simulink model "ToySystem"  (R2019b)
settings: Solver=VariableStepAuto  StartTime=0.0  StopTime=10.0  RelTol=1e-3
undefined symbols (not defined in the file or in its folder): b1, b2, Cp_wall, D, dH, dH1, dH2, f, f1, f2, Fluid, Fluid1, Fluid2, H, HTC, HTC1, HTC2, HTC_method, HTC_method1, HTC_method2, KL, KL1, KL2, L, L1, L2, M_wall, Nu_lam1, Nu_lam2, P_init, PAF, Pamb, Pass1, Pass2, rev_comms_sink, Tw_init, v, W1, W2
libraries: DAEMOT_Lib x21
(part 1 of 2)
settings Model: Creator=aksland2  LastModifiedBy=aksland2

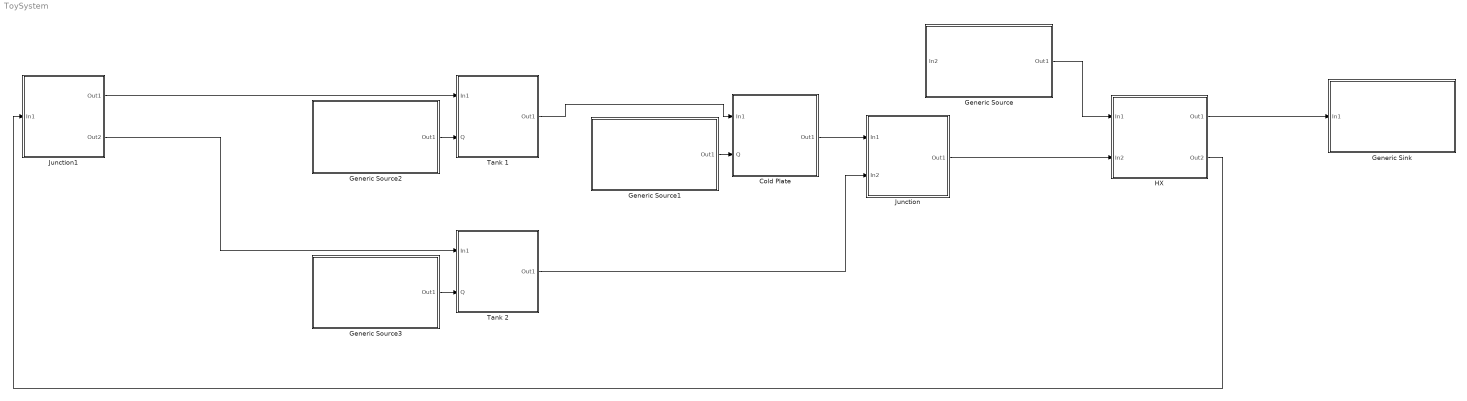
== system ToySystem ==
  Cold Plate : Subsystem  AncestorBlock=DAEMOT_Lib/Thermal/Cold_Plate  mask(Cold Plate){fluid=PG50, P_init=113, T_init=20, cp_f=4000}
      mask prompts: fluid "Fluid Type"; P_init "Initial Outlet Pressure [kPa]"; T_init "Initial Outlet Temperature [°C]"; cp_f "Specific Head"
      mask help: Tracks the time rate of change of the pressure, wall temperature, and fluid exit temperature.
      mask init:
      | % load('Fluids.mat');
      | % Fluid = eval(['Fluid.',fld]);
      | % 
      | % load('Moody.mat');
      settings: OpenFcn=|
      | load('Fluids.mat');
      | Set_Fluid_Popup_Names( Fluid )
      mask TypeOptions fluid: Fuel | Water | Air | PG50
      mask DialogControl Container5 Prompt: Parameters
      mask Display:
      | image(imread('ColdPlate.jpg'))
      | 
      | text(0.5,0.95,['{\bf ',fluid,' Cold Plate}'],'TexMode','on','horizontalAlignment', 'center')
      | text(0.5,0.08,['{-----(P)}'],'TexMode','on','horizontalAlignment', 'center')
      | 
      | port_label('input',1,'Flow In')
      | port_label('input',2,'Thermal In')
      | port_label('output',1,'Flow Out')
  Generic Sink : Subsystem  AncestorBlock=DAEMOT_Lib/Support Functions/Generic Sink  mask(Effort Sink (Torque)){Stype=Mass Flow Sink, const=on, value=0}
      mask prompts: Stype "Sink Type"; const "Constant Value?"; value "Mass Flow [kg/s]"
      mask help: Used to create a effot sink.
      mask init:
      | h      = get_param(gcb,'handle');   % Get block handle
      | blk    = gcb;
      | hblock = get(h);     % Parse out handles structure
      | 
      | if const == 1;
      |     try delete_block([blk,'/In2'])
      |         delete_unconnected_lines(blk);
      |         add_block('simulink/Sources/Constant',   [blk,'/val'], 'Position', [200,218,230,232]);
      |         add_line(blk,'val/1','Sink1/1','AutoRouting','on');
      |         set_param([blk,'/val'],'Value','value');
      |     end
      |      
      | %     delete_unconnected_lines(blk)
      | else
      |     try delete_block([blk,'/val'])
      |         delete_unconnected_lines(blk);
      |         add_block('simulink/Ports & Subsystems/In1',   [blk,'/In2'], 'Position', [200,218,230,232]);
      |         add_line(blk,'In2/1','Sink1/1','AutoRouting','on');
      |     end
      | end
      | 
      | clear h blk hblock
      settings: CopyFcn=|
      | h      = get_param(gcb,'handle');   % Get block handle
      | blk    = gcb;
      | 
      | set_param(blk, 'LinkStatus', 'inactive')
      | clear h
      | clear blk
      mask TypeOptions Stype: Voltage Sink | Current Sink | Angular Speed Sink | Torque Sink | Temperature Sink | Heat Flow Sink | Pressure Sink | Mass Flow Sink
      mask Callback Stype:
      | mp     = get_param(gcb,'MaskPrompts');
      | h      = get_param(gcb,'handle');   % Get block handle
      | blk    = gcb;
      | hblock = get(h);     % Parse out handles structure
      | 
      | switch get_param(gcb,'Stype')
      |     case 'Voltage Sink'
      |         mp{3} = 'Voltage [V]';
      |     case 'Current Sink'
      |         mp{3} = 'Current [A]';
      |     case 'Angular Speed Sink'
      |         mp{3} = 'Speed [rad/s]';
      |     case 'Torque Sink'
      |         mp{3} = 'Torque [Nm]';
      |     case 'Temperature Sink'
      |         mp{3} = 'Temperature [C]';
      |     case 'Heat Flow Sink'
      |         mp{3} = 'Heat Flow [kW]';
      |     case 'Pressure Sink'
      |         mp{3} = 'Pressure [kPa]';
      |     case 'Mass Flow Sink'
      |         mp{3} = 'Mass Flow [kg/s]';
      | end
      | set_param(gcb,'MaskPrompts',mp);
      | 
      | clear mp h blk hblock
      mask Callback const:
      | en = get_param(gcb,'MaskVisibilities');
      | h      = get_param(gcb,'handle');   % Get block handle
      | blk    = gcb;
      | hblock = get(h);     % Parse out handles structure
      | 
      | switch get_param(gcb,'const')
      |     case 'on'
      |         en{3} = 'on';
      | %         delete_block([blk,'/In1'])
      | 
      |     case 'off'
      |         en{3} = 'off';
      | %         add_block('simulink/Ports & Subsystems/In1',   [blk,'/In1'],'Position',[130    -7   160     7]);         % adding inport
      | 
      | end
      | set_param(gcb,'MaskVisibilities',en);
      | 
      | % hblock.MaskPrompts{3} = 'hello';
      | clear en h blk hblock
      mask Display:
      | text(0.5,0.90,['{\bf',get_param(gcb,'Stype'),'}'],'TexMode','on','horizontalAlignment', 'center')
      | % text(0.5,0.1,['{(T)(end)}'],'TexMode','on','horizontalAlignment', 'center')
      | 
      | type = get_param(gcb,'Stype');
      | switch type
      |         case 'Voltage Sink'
      |             nm = 'Voltage [V]';
      |             id = '(V)';
      |             un = 'V';
      |         case 'Current Sink'
      |             nm = 'Current [A]';
      |             id = '(----)';
      |             un = 'A';
      |         case 'Angular Speed Sink'
      |             nm = 'Speed [rad/s]';
      |             id = '(----)';
      |             un = 'rad/s';
      |         case 'Torque Sink'
      |             nm = 'Torque [Nm]';
      |             id = '(\tau)';
      |             un = 'Nm';
      |         case 'Temperature Sink'
      |             nm = 'Temperature [C]';
      |             id = '(T)';
      |             un = 'C';
      |         case 'Heat Flow Sink'
      |             nm = 'Heat Flow [kW]';
      |             id = '(----)';
      |             un = 'kW';
      |         case 'Pressure Sink'
      |             nm = 'Pressure [kPa]';
      |             id = '(P)';
      |             un = 'kPa';
      |         case 'Mass Flow Sink'
      |             nm = 'Mass Flow [kg/s]';
      |             id = '(----)';
      |             un = 'kg/s';
      | end
      | 
      | if strcmp(get_param(gcb,'const'),'on')
      |     text(0.75,0.500,['{\bf',get_param(gcb,'Value'),un,'}'],'TexMode','on','horizontalAlignment', 'center')
      | else
      |     port_label('input',2,sprintf(['Sink ',nm]));
      | end
      | 
      | 
      | port_label('input',1,'Sink');
      | text(0.5,0.175,['{',id,' (end)}'],'TexMode','on','horizontalAlignment', 'center');
  Generic Source : Subsystem  AncestorBlock=DAEMOT_Lib/Support Functions/Generic Source  mask(Effort Source (Voltage)){Stype=Pressure Source, const=on, value=0}
      mask prompts: Stype "Source Type"; const "Constant Value?"; value "Pressure [kPa]"
      mask help: Used to create an effort source.
      mask init:
      | h      = get_param(gcb,'handle');   % Get block handle
      | blk    = gcb;
      | hblock = get(h);     % Parse out handles structure
      | type = get_param(gcb,'Stype');
      |         
      | switch type
      |     case 'Voltage Source'
      |         up = 'current';
      |         dw = 'voltage';
      |     case 'Current Source'
      |         dw = 'current';
      |         up = 'voltage';
      |     case 'Angular Speed Source'
      |         up = 'torque';
      |         dw = 'aspeed';
      |     case 'Torque Source'
      |         dw = 'torque';
      |         up = 'aspeed';
      |     case 'Temperature Source'
      |         up = 'Q_kW';
      |         dw = 'Temp';
      |     case 'Heat Flow Source'
      |         dw = 'Q_kW';
      |         up = 'Temp';
      |     case 'Pressure Source'
      |         up = 'mdot_kgps';
      |         mid= 'T_C';
      |         dw = 'P_kPa';
      |     case 'Mass Flow Source'
      |         up = 'mdot_kgps';
      |         mid= 'T_C';
      |         dw = 'P_kPa';
      | end
      | 
      | if (((type(1) == 'P') || (type(1) == 'M')) && (const == 1)) %if constant input (user defined in mask) and need temperature input
      |     
      |     try add_block('simulink/Ports & Subsystems/In1', [blk,'/In2'], 'Position', [200,230,230,245]) %make temperature input
      |         set_param([blk, '/b1'],'Inputs','3');
      |         add_line(blk,'In2/1','b1/3','AutoRouting','on');
      |             
      |         p = get_param([blk,'/In2'],'PortHandles');
      |         l = get_param(p.Outport,'Line');
      |         set_param(l,'Name',mid);
      |     end 
      |     
      |     try delete_block([blk,'/In1'])
      |         delete_unconnected_lines(blk);
      |         
      |         fprintf ("option 1\n");        
      |         
      |         add_block('simulink/Sources/Constant',   [blk,'/val'], 'Position', [200,148,230,162]);
      |         add_line(blk,'val/1','b1/2','AutoRouting','on');
      |         set_param([blk,'/val'],'Value','value');
      |         
      |         p = get_param([blk,'/Constant'],'PortHandles');
      |         l = get_param(p.Outport,'Line');
      |         set_param(l,'Name',up);
      | 
      |         p = get_param([blk,'/val'],'PortHandles');
      |         l = get_param(p.Outport,'Line');
      |         set_param(l,'Name',dw);
      |         
      |     end
      |     p = get_param([blk,'/Constant'],'PortHandles');
      |     l = get_param(p.Outport,'Line');
      | 
      |     if (strcmp(get_param(l,'name'),up)) %If it didn't work and l's name doesn't match what it should, set them again.
      |     else
      |         set_param(l,'Name',up);
      |         
      |         fprintf ("failed strcmp \n");
      |                 
      |         p = get_param([blk,'/val'],'PortHandles');
      |         l = get_param(p.Outport,'Line');
      |         set_param(l,'Name',dw);
      |             
      |         p = get_param([blk,'/In2'],'PortHandles');
      |         l = get_param(p.Outport,'Line');
      |         set_param(l,'Name',mid);
      |     end
      |     
      | elseif ((type(1) == 'P') || (type(1) == 'M')) %if need input port (not user defined in mask) and also need temperature input
      |     
      |     try add_block('simulink/Ports & Subsystems/In1', [blk,'/In2'], 'Position', [200,230,230,245]) %make temperature input
      |         set_param([blk, '/b1'],'Inputs','3');
      |         add_line(blk,'In2/1','b1/3','AutoRouting','on');
      | 
      |         p = get_param([blk,'/In2'],'PortHandles');
      |         l = get_param(p.Outport,'Line');
      |         set_param(l,'Name',mid);
      |     end
      |     
      |     try delete_block([blk,'/val'])
      |         delete_unconnected_lines(blk);
      |         
      |         fprintf ("option 2\n");      
      |         
      |         add_block('simulink/Ports & Subsystems/In1', [blk,'/In1'], 'Position', [200,148,230,162]);
      |         add_line(blk,'In1/1','b1/2','AutoRouting','on');
      |         
      |         p = get_param([blk,'/Constant'],'PortHandles');
      |         l = get_param(p.Outport,'Line');
      |         set_param(l,'Name',up);
      | 
      |         p = get_param([blk,'/In1'],'PortHandles');
      |         l = get_param(p.Outport,'Line');
      |         set_param(l,'Name',dw);
      |         
      |     end
      |     
      |     p = get_param([blk,'/Constant'],'PortHandles');
      |     l = get_param(p.Outport,'Line');
      |     if (strcmp(get_param(l,'name'),up)) %If it didn't work and l's name doesn't match what it should, set them again.
      |     else
      |         set_param(l,'Name',up);
      |         
      |         fprintf ("failed strcmp \n");
      |         
      |         p = get_param([blk,'/In1'],'PortHandles');
      |         l = get_param(p.Outport,'Line');
      |         set_param(l,'Name',dw);
      | 
      |         p = get_param([blk,'/In2'],'PortHandles');
      |         l = get_param(p.Outport,'Line');
      |         set_param(l,'Name',mid);
      |     end
      |     
      | elseif (const == 1) %if constant, user-defined input, but does not need a temperature input port
      |     try delete_block([blk,'/In2']) %delete temperature input
      |         delete_unconnected_lines(blk);
      |         
      |         set_param([blk, '/b1'],'Inputs','2');
      |         fprintf ("delete in2 \n");
      |     end
      |     
      |     try delete_block([blk,'/In1'])
      |         delete_unconnected_lines(blk);
      |         
      |         fprintf ("option 3\n");
      |         
      |         add_block('simulink/Sources/Constant',   [blk,'/val'], 'Position', [200,198,230,212]);
      |         add_line(blk,'val/1','b1/2','AutoRouting','on');
      |         set_param([blk,'/val'],'Value','value');
      |         
      |         p = get_param([blk,'/Constant'],'PortHandles');
      |         l = get_param(p.Outport,'Line');
      |         set_param(l,'Name',up);
      |         
      |         p = get_param([blk,'/val'],'PortHandles');
      |         l = get_param(p.Outport,'Line');
      |         set_param(l,'Name',dw);
      |     end
      |     
      |     p = get_param([blk,'/Constant'],'PortHandles');
      |     l = get_param(p.Outport,'Line');
      |     if (strcmp(get_param(l,'name'),up))
      |     else
      |         set_param(l,'Name',up);
      |         
      |         fprintf ("failed strcmp \n");
      |                 
      |         p = get_param([blk,'/val'],'PortHandles');
      |         l = get_param(p.Outport,'Line');
      |         set_param(l,'Name',dw);
      |     end
      |     
      | else %if need an input port for the input, but not for temperature
      |     try delete_block([blk,'/In2']) %delete temperature input
      |         delete_unconnected_lines(blk);
      |         
      |         set_param([blk, '/b1'],'Inputs','2');
      |         fprintf ("deleted in2 \n");
      |     end    
      |         
      |     try delete_block([blk,'/val'])
      |         delete_unconnected_lines(blk);
      |         
      |         fprintf ("option 4\n");
      |         
      |         add_block('simulink/Ports & Subsystems/In1',   [blk,'/In1'], 'Position', [200,198,230,212]);
      |         add_line(blk,'In1/1','b1/2','AutoRouting','on');
      |         
      |         p = get_param([blk,'/Constant'],'PortHandles');
      |         l = get_param(p.Outport,'Line');
      |         set_param(l,'Name',up);
      | 
      |         p = get_param([blk,'/In1'],'PortHandles');
      |         l = get_param(p.Outport,'Line');
      |         set_param(l,'Name',dw);
      |     end
      |     
      |     p = get_param([blk,'/Constant'],'PortHandles');
      |     l = get_param(p.Outport,'Line');
      |     if (strcmp(get_param(l,'name'),up))
      |     else
      |         set_param(l,'Name',up);
      |         fprintf ("failed strcmp \n");
      |         p = get_param([blk,'/In1'],'PortHandles');
      |         l = get_param(p.Outport,'Line');
      |         set_param(l,'Name',dw);
      |     end
      |     
      | end
      | 
      | 
      | %if const == 1;
      | %    try delete_block([blk,'/In1'])
      | %        delete_unconnected_lines(blk);
      | %        add_block('simulink/Sources/Constant',   [blk,'/val'], 'Position', [200,198,230,212]);
      | %        add_line(blk,'val/1','b1/2','AutoRouting','on');
      | %        set_param([blk,'/val'],'Value','value');
      | 
      | %        p = get_param([blk,'/Constant'],'PortHandles');
      | %        l = get_param(p.Outport,'Line');
      | %        set_param(l,'Name',up);
      |         
      | %        p = get_param([blk,'/val'],'PortHandles');
      | %        l = get_param(p.Outport,'Line');
      | %        set_param(l,'Name',dw);
      | %    end
      | %    p = get_param([blk,'/Constant'],'PortHandles');
      | %    l = get_param(p.Outport,'Line');
      | %    if strcmp(get_param(l,'name'),up)
      | %    else
      | %       set_param(l,'Name',up);
      |         
      | %        p = get_param([blk,'/val'],'PortHandles');
      | %        l = get_param(p.Outport,'Line');
      | %        set_param(l,'Name',dw);
      | %    end
      |      
      | %%     delete_unconnected_lines(blk)
      | %else
      | %    try delete_block([blk,'/val'])
      | %        delete_unconnected_lines(blk);
      | %        add_block('simulink/Ports & Subsystems/In1',   [blk,'/In1'], 'Position', [200,198,230,212]);
      | %        add_line(blk,'In1/1','b1/2','AutoRouting','on');
      |         
      | %        p = get_param([blk,'/Constant'],'PortHandles');
      | %        l = get_param(p.Outport,'Line');
      | %        set_param(l,'Name',up);
      | 
      | %        p = get_param([blk,'/In1'],'PortHandles');
      | %        l = get_param(p.Outport,'Line');
      | %        set_param(l,'Name',dw);
      | %    end
      | %    p = get_param([blk,'/Constant'],'PortHandles');
      | %    l = get_param(p.Outport,'Line');
      | %    if strcmp(get_param(l,'name'),up)
      | %    else
      | %        set_param(l,'Name',up);
      |         
      | %        p = get_param([blk,'/In1'],'PortHandles');
      | %        l = get_param(p.Outport,'Line');
      | %        set_param(l,'Name',dw);
      | %    end
      | %end
      | 
      | clear h blk hblock type
      settings: CopyFcn=|
      | h      = get_param(gcb,'handle');   % Get block handle
      | blk    = gcb;
      | 
      | set_param(blk, 'LinkStatus', 'inactive')
      | clear h
      | clear blk
      mask TypeOptions Stype: Voltage Source | Current Source | Angular Speed Source | Torque Source | Temperature Source | Heat Flow Source | Pressure Source | Mass Flow Source
      mask Callback Stype:
      | mp     = get_param(gcb,'MaskPrompts');
      | h      = get_param(gcb,'handle');   % Get block handle
      | blk    = gcb;
      | hblock = get(h);     % Parse out handles structure
      | 
      | switch get_param(gcb,'Stype')
      |     case 'Voltage Source'
      |         mp{3} = 'Voltage [V]';
      |     case 'Current Source'
      |         mp{3} = 'Current [A]';
      |     case 'Angular Speed Source'
      |         mp{3} = 'Speed [rad/s]';
      |     case 'Torque Source'
      |         mp{3} = 'Torque [Nm]';
      |     case 'Temperature Source'
      |         mp{3} = 'Temperature [C]';
      |     case 'Heat Flow Source'
      |         mp{3} = 'Heat Flow [kW]';
      |     case 'Pressure Source'
      |         mp{3} = 'Pressure [kPa]';
      |     case 'Mass Flow Source'
      |         mp{3} = 'Mass Flow [kg/s]';
      | end
      | set_param(gcb,'MaskPrompts',mp);
      | 
      | clear mp h blk hblock
      mask Callback const:
      | en = get_param(gcb,'MaskVisibilities');
      | h      = get_param(gcb,'handle');   % Get block handle
      | blk    = gcb;
      | hblock = get(h);     % Parse out handles structure
      | 
      | switch get_param(gcb,'const')
      |     case 'on'
      |         en{3} = 'on';
      | %         delete_block([blk,'/In1'])
      | 
      |     case 'off'
      |         en{3} = 'off';
      | %         add_block('simulink/Ports & Subsystems/In1',   [blk,'/In1'],'Position',[130    -7   160     7]);         % adding inport
      | 
      | end
      | set_param(gcb,'MaskVisibilities',en);
      | 
      | % hblock.MaskPrompts{3} = 'hello';
      | clear en h blk hblock
      mask Display:
      | text(0.5,0.900,['{\bf',get_param(gcb,'Stype'),'}'],'TexMode','on','horizontalAlignment', 'center')
      | 
      | type = get_param(gcb,'Stype');
      | switch type
      |     case 'Voltage Source'
      |         nm = 'Voltage [V]';
      |         id = '(V)*';
      |         un = 'V';
      |     case 'Current Source'
      |         nm = 'Current [A]';
      |         id = '(----)';
      |         un = 'A';
      |     case 'Angular Speed Source'
      |         nm = 'Speed [rad/s]';
      |         id = '(----)';
      |         un = 'rad/s';
      |     case 'Torque Source'
      |         nm = 'Torque [Nm]';
      |         id = '(\tau)*';
      |         un = 'Nm';
      |     case 'Temperature Source'
      |         nm = 'Temperature [C]';
      |         id = '(T)';
      |         un = 'C';
      |     case 'Heat Flow Source'
      |         nm = 'Heat Flow [kW]';
      |         id = '(----)';
      |         un = 'kW';
      |     case 'Pressure Source'
      |         nm = 'Pressure [kPa]';
      |         id = '(P)';
      |         un = 'kPa';
      |     case 'Mass Flow Source'
      |         nm = 'Mass Flow [kg/s]';
      |         id = '(----)';
      |         un = 'kg/s';
      | end
      | 
      | if strcmp(get_param(gcb,'const'),'on')
      |     text(0.35,0.500,['{\bf',get_param(gcb,'Value'),un,'}'],'TexMode','on','horizontalAlignment', 'center')
      | else
      |     port_label('input',1,sprintf(['Source \n',nm]))
      | end
      | port_label('output',1,'Source')
      | text(0.5,0.175,['{(start) ',id,'}'],'TexMode','on','horizontalAlignment', 'center')
      | 
      | switch type
      |     case 'Pressure Source'
      |         if strcmp(get_param(gcb,'const'),'off')
      |             port_label('input',2,sprintf(['Source\nTemp. [C]']))
      |         else
      |             port_label('input',1,sprintf(['Source\nTemp. [C]']))
      | 
      |         end
      |     case 'Mass Flow Source'
      |         if strcmp(get_param(gcb,'const'),'off')
      |             port_label('input',2,sprintf(['Source\nTemp. [C]']))
      |         else
      |             port_label('input',1,sprintf(['Source\nTemp. [C]']))
      | 
      |         end
      | end
  Generic Source1 : Subsystem  AncestorBlock=DAEMOT_Lib/Support Functions/Generic Source  mask(Effort Source (Voltage)){Stype=Heat Flow Source, const=on, value=0}
      mask prompts: Stype "Source Type"; const "Constant Value?"; value "Heat Flow [kW]"
      mask help: Used to create an effort source.
      mask init: same as ToySystem/Generic Source
      settings: CopyFcn=|
      | h      = get_param(gcb,'handle');   % Get block handle
      | blk    = gcb;
      | 
      | set_param(blk, 'LinkStatus', 'inactive')
      | clear h
      | clear blk
      mask TypeOptions Stype: Voltage Source | Current Source | Angular Speed Source | Torque Source | Temperature Source | Heat Flow Source | Pressure Source | Mass Flow Source
      mask Callback Stype:
      | mp     = get_param(gcb,'MaskPrompts');
      | h      = get_param(gcb,'handle');   % Get block handle
      | blk    = gcb;
      | hblock = get(h);     % Parse out handles structure
      | 
      | switch get_param(gcb,'Stype')
      |     case 'Voltage Source'
      |         mp{3} = 'Voltage [V]';
      |     case 'Current Source'
      |         mp{3} = 'Current [A]';
      |     case 'Angular Speed Source'
      |         mp{3} = 'Speed [rad/s]';
      |     case 'Torque Source'
      |         mp{3} = 'Torque [Nm]';
      |     case 'Temperature Source'
      |         mp{3} = 'Temperature [C]';
      |     case 'Heat Flow Source'
      |         mp{3} = 'Heat Flow [kW]';
      |     case 'Pressure Source'
      |         mp{3} = 'Pressure [kPa]';
      |     case 'Mass Flow Source'
      |         mp{3} = 'Mass Flow [kg/s]';
      | end
      | set_param(gcb,'MaskPrompts',mp);
      | 
      | clear mp h blk hblock
      mask Callback const:
      | en = get_param(gcb,'MaskVisibilities');
      | h      = get_param(gcb,'handle');   % Get block handle
      | blk    = gcb;
      | hblock = get(h);     % Parse out handles structure
      | 
      | switch get_param(gcb,'const')
      |     case 'on'
      |         en{3} = 'on';
      | %         delete_block([blk,'/In1'])
      | 
      |     case 'off'
      |         en{3} = 'off';
      | %         add_block('simulink/Ports & Subsystems/In1',   [blk,'/In1'],'Position',[130    -7   160     7]);         % adding inport
      | 
      | end
      | set_param(gcb,'MaskVisibilities',en);
      | 
      | % hblock.MaskPrompts{3} = 'hello';
      | clear en h blk hblock
      mask Display:
      | text(0.5,0.900,['{\bf',get_param(gcb,'Stype'),'}'],'TexMode','on','horizontalAlignment', 'center')
      | 
      | type = get_param(gcb,'Stype');
      | switch type
      |     case 'Voltage Source'
      |         nm = 'Voltage [V]';
      |         id = '(V)*';
      |         un = 'V';
      |     case 'Current Source'
      |         nm = 'Current [A]';
      |         id = '(----)';
      |         un = 'A';
      |     case 'Angular Speed Source'
      |         nm = 'Speed [rad/s]';
      |         id = '(----)';
      |         un = 'rad/s';
      |     case 'Torque Source'
      |         nm = 'Torque [Nm]';
      |         id = '(\tau)*';
      |         un = 'Nm';
      |     case 'Temperature Source'
      |         nm = 'Temperature [C]';
      |         id = '(T)';
      |         un = 'C';
      |     case 'Heat Flow Source'
      |         nm = 'Heat Flow [kW]';
      |         id = '(----)';
      |         un = 'kW';
      |     case 'Pressure Source'
      |         nm = 'Pressure [kPa]';
      |         id = '(P)';
      |         un = 'kPa';
      |     case 'Mass Flow Source'
      |         nm = 'Mass Flow [kg/s]';
      |         id = '(----)';
      |         un = 'kg/s';
      | end
      | 
      | if strcmp(get_param(gcb,'const'),'on')
      |     text(0.35,0.500,['{\bf',get_param(gcb,'Value'),un,'}'],'TexMode','on','horizontalAlignment', 'center')
      | else
      |     port_label('input',1,sprintf(['Source \n',nm]))
      | end
      | port_label('output',1,'Source')
      | text(0.5,0.175,['{(start) ',id,'}'],'TexMode','on','horizontalAlignment', 'center')
      | 
      | switch type
      |     case 'Pressure Source'
      |         if strcmp(get_param(gcb,'const'),'off')
      |             port_label('input',2,sprintf(['Source\nTemp. [C]']))
      |         else
      |             port_label('input',1,sprintf(['Source\nTemp. [C]']))
      | 
      |         end
      |     case 'Mass Flow Source'
      |         if strcmp(get_param(gcb,'const'),'off')
      |             port_label('input',2,sprintf(['Source\nTemp. [C]']))
      |         else
      |             port_label('input',1,sprintf(['Source\nTemp. [C]']))
      | 
      |         end
      | end
  Generic Source2 : Subsystem  AncestorBlock=DAEMOT_Lib/Support Functions/Generic Source  mask(Effort Source (Voltage)){Stype=Heat Flow Source, const=on, value=0}
      mask prompts: Stype "Source Type"; const "Constant Value?"; value "Heat Flow [kW]"
      mask help: Used to create an effort source.
      mask init: same as ToySystem/Generic Source
      settings: CopyFcn=|
      | h      = get_param(gcb,'handle');   % Get block handle
      | blk    = gcb;
      | 
      | set_param(blk, 'LinkStatus', 'inactive')
      | clear h
      | clear blk
      mask TypeOptions Stype: Voltage Source | Current Source | Angular Speed Source | Torque Source | Temperature Source | Heat Flow Source | Pressure Source | Mass Flow Source
      mask Callback Stype:
      | mp     = get_param(gcb,'MaskPrompts');
      | h      = get_param(gcb,'handle');   % Get block handle
      | blk    = gcb;
      | hblock = get(h);     % Parse out handles structure
      | 
      | switch get_param(gcb,'Stype')
      |     case 'Voltage Source'
      |         mp{3} = 'Voltage [V]';
      |     case 'Current Source'
      |         mp{3} = 'Current [A]';
      |     case 'Angular Speed Source'
      |         mp{3} = 'Speed [rad/s]';
      |     case 'Torque Source'
      |         mp{3} = 'Torque [Nm]';
      |     case 'Temperature Source'
      |         mp{3} = 'Temperature [C]';
      |     case 'Heat Flow Source'
      |         mp{3} = 'Heat Flow [kW]';
      |     case 'Pressure Source'
      |         mp{3} = 'Pressure [kPa]';
      |     case 'Mass Flow Source'
      |         mp{3} = 'Mass Flow [kg/s]';
      | end
      | set_param(gcb,'MaskPrompts',mp);
      | 
      | clear mp h blk hblock
      mask Callback const:
      | en = get_param(gcb,'MaskVisibilities');
      | h      = get_param(gcb,'handle');   % Get block handle
      | blk    = gcb;
      | hblock = get(h);     % Parse out handles structure
      | 
      | switch get_param(gcb,'const')
      |     case 'on'
      |         en{3} = 'on';
      | %         delete_block([blk,'/In1'])
      | 
      |     case 'off'
      |         en{3} = 'off';
      | %         add_block('simulink/Ports & Subsystems/In1',   [blk,'/In1'],'Position',[130    -7   160     7]);         % adding inport
      | 
      | end
      | set_param(gcb,'MaskVisibilities',en);
      | 
      | % hblock.MaskPrompts{3} = 'hello';
      | clear en h blk hblock
      mask Display:
      | text(0.5,0.900,['{\bf',get_param(gcb,'Stype'),'}'],'TexMode','on','horizontalAlignment', 'center')
      | 
      | type = get_param(gcb,'Stype');
      | switch type
      |     case 'Voltage Source'
      |         nm = 'Voltage [V]';
      |         id = '(V)*';
      |         un = 'V';
      |     case 'Current Source'
      |         nm = 'Current [A]';
      |         id = '(----)';
      |         un = 'A';
      |     case 'Angular Speed Source'
      |         nm = 'Speed [rad/s]';
      |         id = '(----)';
      |         un = 'rad/s';
      |     case 'Torque Source'
      |         nm = 'Torque [Nm]';
      |         id = '(\tau)*';
      |         un = 'Nm';
      |     case 'Temperature Source'
      |         nm = 'Temperature [C]';
      |         id = '(T)';
      |         un = 'C';
      |     case 'Heat Flow Source'
      |         nm = 'Heat Flow [kW]';
      |         id = '(----)';
      |         un = 'kW';
      |     case 'Pressure Source'
      |         nm = 'Pressure [kPa]';
      |         id = '(P)';
      |         un = 'kPa';
      |     case 'Mass Flow Source'
      |         nm = 'Mass Flow [kg/s]';
      |         id = '(----)';
      |         un = 'kg/s';
      | end
      | 
      | if strcmp(get_param(gcb,'const'),'on')
      |     text(0.35,0.500,['{\bf',get_param(gcb,'Value'),un,'}'],'TexMode','on','horizontalAlignment', 'center')
      | else
      |     port_label('input',1,sprintf(['Source \n',nm]))
      | end
      | port_label('output',1,'Source')
      | text(0.5,0.175,['{(start) ',id,'}'],'TexMode','on','horizontalAlignment', 'center')
      | 
      | switch type
      |     case 'Pressure Source'
      |         if strcmp(get_param(gcb,'const'),'off')
      |             port_label('input',2,sprintf(['Source\nTemp. [C]']))
      |         else
      |             port_label('input',1,sprintf(['Source\nTemp. [C]']))
      | 
      |         end
      |     case 'Mass Flow Source'
      |         if strcmp(get_param(gcb,'const'),'off')
      |             port_label('input',2,sprintf(['Source\nTemp. [C]']))
      |         else
      |             port_label('input',1,sprintf(['Source\nTemp. [C]']))
      | 
      |         end
      | end
  Generic Source3 : Subsystem  AncestorBlock=DAEMOT_Lib/Support Functions/Generic Source  mask(Effort Source (Voltage)){Stype=Heat Flow Source, const=on, value=0}
      mask prompts: Stype "Source Type"; const "Constant Value?"; value "Heat Flow [kW]"
      mask help: Used to create an effort source.
      mask init: same as ToySystem/Generic Source
      settings: CopyFcn=|
      | h      = get_param(gcb,'handle');   % Get block handle
      | blk    = gcb;
      | 
      | set_param(blk, 'LinkStatus', 'inactive')
      | clear h
      | clear blk
      mask TypeOptions Stype: Voltage Source | Current Source | Angular Speed Source | Torque Source | Temperature Source | Heat Flow Source | Pressure Source | Mass Flow Source
      mask Callback Stype:
      | mp     = get_param(gcb,'MaskPrompts');
      | h      = get_param(gcb,'handle');   % Get block handle
      | blk    = gcb;
      | hblock = get(h);     % Parse out handles structure
      | 
      | switch get_param(gcb,'Stype')
      |     case 'Voltage Source'
      |         mp{3} = 'Voltage [V]';
      |     case 'Current Source'
      |         mp{3} = 'Current [A]';
      |     case 'Angular Speed Source'
      |         mp{3} = 'Speed [rad/s]';
      |     case 'Torque Source'
      |         mp{3} = 'Torque [Nm]';
      |     case 'Temperature Source'
      |         mp{3} = 'Temperature [C]';
      |     case 'Heat Flow Source'
      |         mp{3} = 'Heat Flow [kW]';
      |     case 'Pressure Source'
      |         mp{3} = 'Pressure [kPa]';
      |     case 'Mass Flow Source'
      |         mp{3} = 'Mass Flow [kg/s]';
      | end
      | set_param(gcb,'MaskPrompts',mp);
      | 
      | clear mp h blk hblock
      mask Callback const:
      | en = get_param(gcb,'MaskVisibilities');
      | h      = get_param(gcb,'handle');   % Get block handle
      | blk    = gcb;
      | hblock = get(h);     % Parse out handles structure
      | 
      | switch get_param(gcb,'const')
      |     case 'on'
      |         en{3} = 'on';
      | %         delete_block([blk,'/In1'])
      | 
      |     case 'off'
      |         en{3} = 'off';
      | %         add_block('simulink/Ports & Subsystems/In1',   [blk,'/In1'],'Position',[130    -7   160     7]);         % adding inport
      | 
      | end
      | set_param(gcb,'MaskVisibilities',en);
      | 
      | % hblock.MaskPrompts{3} = 'hello';
      | clear en h blk hblock
      mask Display:
      | text(0.5,0.900,['{\bf',get_param(gcb,'Stype'),'}'],'TexMode','on','horizontalAlignment', 'center')
      | 
      | type = get_param(gcb,'Stype');
      | switch type
      |     case 'Voltage Source'
      |         nm = 'Voltage [V]';
      |         id = '(V)*';
      |         un = 'V';
      |     case 'Current Source'
      |         nm = 'Current [A]';
      |         id = '(----)';
      |         un = 'A';
      |     case 'Angular Speed Source'
      |         nm = 'Speed [rad/s]';
      |         id = '(----)';
      |         un = 'rad/s';
      |     case 'Torque Source'
      |         nm = 'Torque [Nm]';
      |         id = '(\tau)*';
      |         un = 'Nm';
      |     case 'Temperature Source'
      |         nm = 'Temperature [C]';
      |         id = '(T)';
      |         un = 'C';
      |     case 'Heat Flow Source'
      |         nm = 'Heat Flow [kW]';
      |         id = '(----)';
      |         un = 'kW';
      |     case 'Pressure Source'
      |         nm = 'Pressure [kPa]';
      |         id = '(P)';
      |         un = 'kPa';
      |     case 'Mass Flow Source'
      |         nm = 'Mass Flow [kg/s]';
      |         id = '(----)';
      |         un = 'kg/s';
      | end
      | 
      | if strcmp(get_param(gcb,'const'),'on')
      |     text(0.35,0.500,['{\bf',get_param(gcb,'Value'),un,'}'],'TexMode','on','horizontalAlignment', 'center')
      | else
      |     port_label('input',1,sprintf(['Source \n',nm]))
      | end
      | port_label('output',1,'Source')
      | text(0.5,0.175,['{(start) ',id,'}'],'TexMode','on','horizontalAlignment', 'center')
      | 
      | switch type
      |     case 'Pressure Source'
      |         if strcmp(get_param(gcb,'const'),'off')
      |             port_label('input',2,sprintf(['Source\nTemp. [C]']))
      |         else
      |             port_label('input',1,sprintf(['Source\nTemp. [C]']))
      | 
      |         end
      |     case 'Mass Flow Source'
      |         if strcmp(get_param(gcb,'const'),'off')
      |             port_label('input',2,sprintf(['Source\nTemp. [C]']))
      |         else
      |             port_label('input',1,sprintf(['Source\nTemp. [C]']))
      | 
      |         end
      | end
  HX : Subsystem  AncestorBlock=DAEMOT_Lib/Thermal/Heat Exchanger  mask(Heat Exchanger){Tw_init=22, fluid1=PG50, P1_init=110, T1_init=22, cp_f1=0.05, fluid2=PG50, P2_init=110, T2_init=22, cp_f2=0.05}
      mask prompts: Tw_init "Initial Wall Temperature [°C]"; fluid1 "Fluid Type 1"; P1_init "Initial Outlet 1 Pressure [kPa]"; T1_init "Initial Outlet 1 Temperature [°C]"; cp_f1 "Specfic Heat"; fluid2 "Fluid Type 2"; P2_init "Initial Outlet 2 Pressure [kPa]"; T2_init "Initial Outlet 2 Temperature [°C]"; cp_f2 "Specfic Heat"
      mask help: Tracks the time rate of change of the pressure, wall temperature, and exit flow temperatures.
      mask init:
      | % load('Fluids.mat');
      | % Fluid1 = eval(['Fluid.',fld1]);
      | % Fluid2 = eval(['Fluid.',fld2]);
      | % 
      | % load('Moody.mat');
      | % 
      | % load('Laminar_Props.mat')
      | % Nu_lam1 = interp1(LamProps.b_a,LamProps.Nu,max(W1,b1)/min(W1,b1));
      | % Nu_lam2 = interp1(LamProps.b_a,LamProps.Nu,max(W2,b2)/min(W2,b2));
      | % set_param(gcb,'Nu_lam1',num2str(Nu_lam1));
      | % set_param(gcb,'Nu_lam2',num2str(Nu_lam2));
      settings: OpenFcn=|
      | load('Fluids.mat');
      | Set_Fluid_Popup_Names( Fluid )
      mask TypeOptions fluid1: Fuel | Water | Air | PG50
      mask TypeOptions fluid2: Fuel | Water | Air | PG50
      mask DialogControl Container10 Prompt: Parameters
      mask DialogControl Container18 Prompt: Side 1
      mask DialogControl Container17 Prompt: Side 2
      mask Display:
      | image(imread('HX.jpg'))
      | 
      | text(0.5,0.95,['{\bf ',fluid1,'/',fluid2,' HX}'],'TexMode','on','horizontalAlignment', 'center')
      | text(0.5,0.08,['{-----(P)}'],'TexMode','on','horizontalAlignment', 'center')
      | 
      | port_label('input',1,['In 1 (',fluid1,')'])
      | port_label('input',2,['In 2 (',fluid2,')'])
      | port_label('output',1,['Out 1 (',fluid1,')'])
      | port_label('output',2,['Out 2 (',fluid2,')'])
  Junction : Subsystem  AncestorBlock=DAEMOT_Lib/Thermal/Flow Split_Junction  mask(Split/Junction){fluid=PG50, n_out=1, n_in=2, cp_f=110, T_init=22, D=0.013, L=0.1, t=0.0015, E=2.4e6, v=0.4}
      mask prompts: fluid "Fluid Type"; n_out "Number of Outlet Flows"; n_in "Number of Inlet Flows"; cp_f "specific heat"; T_init "Initial Temperature [°C]"; D "Diameter [m]"; L "Length [m]"; t "Tube Wall Thickness [m]"; E "Tube Modulus of Elasticity [kPa]"; v "Tube Poisson Ratio [-]"
      mask help: Splits and junctions flows using dynamic relationships. Note that the library link of the block is disabled when it is imported into a model.
      mask init:
      | h      = get_param(gcb,'handle');   % Get block handle
      | blk    = gcb;
      | hblock = get(h);     % Parse out handles structure
      | 
      | % load('Fluids.mat');
      | % Fluid = eval(['Fluid.',fld]);
      | 
      | % delete any previous inports and bus selectors
      | for i = str2num(hblock.n_in)+1:hblock.Ports(1)
      |     delete_block([blk,'/In',num2str(i)])
      |     delete_block([blk,'/gb',num2str(i)])
      |     delete_block([blk,'/gm',num2str(i)])
      |     delete_block([blk,'/gt',num2str(i)])
      |     delete_block([blk,'/gp',num2str(i)])
      |     delete_block([blk,'/Sink',num2str(i)])
      |     delete_block([blk,'/pout',num2str(i)])
      |     delete_block([blk,'/min',num2str(i)])
      |     delete_block([blk,'/tin',num2str(i)])
      |     
      |     delete_unconnected_lines(blk)
      | end
      | 
      | % delete any previous inports and bus selectors
      | for i = str2num(hblock.n_out)+1:hblock.Ports(2)
      |     delete_block([blk,'/Out',num2str(i)])
      |     delete_block([blk,'/m',num2str(i)])
      |     delete_block([blk,'/t',num2str(i)])
      |     delete_block([blk,'/p',num2str(i)])
      |     delete_block([blk,'/b',num2str(i)])
      |     delete_block([blk,'/Source',num2str(i)])
      |     delete_block([blk,'/g',num2str(i)])
      |     delete_block([blk,'/mout',num2str(i)])
      |     %delete_block([blk,'/tout',num2str(i)])
      |     
      |     delete_unconnected_lines(blk)
      | end
      | 
      | set_param([blk,'/Mux_In_1'],'Inputs',hblock.n_in)
      | set_param([blk,'/Mux_In_2'],'Inputs',hblock.n_out)
      | set_param([blk,'/Mux_In_3'],'Inputs',hblock.n_in)
      | %set_param([blk,'/Mux_Out_1'],'Outputs',hblock.n_out)
      | 
      | % generate inports, bus selectors, and route lines to each vector concat
      | for i = hblock.Ports(1)+1:str2num(hblock.n_in)
      |     
      |     % add blocks
      |     add_block('simulink/Ports & Subsystems/In1',   [blk,'/In',num2str(i)],    'Position',[120 i*80-25+20 150 i*80-12+20]);         % adding inport
      |     add_block([blk,'/gb1'],                        [blk,'/gb',num2str(i)],   'Position',[200 i*80-20+20-18 205 i*80-2+20+2]);         % adding inport
      |     add_block('simulink/Signal Routing/Goto',      [blk,'/gm',num2str(i)],    'Position',[260 i*80-17 340 i*80-3]);         % adding inport
      |     add_block('simulink/Signal Routing/Goto',      [blk,'/gt',num2str(i)],    'Position',[260 i*80+3 340 i*80+17]);         % adding inport
      |     add_block('simulink/Sinks/Terminator',          [blk,'/gp',num2str(i)],    'Position',[260 i*80+23 280 i*80+37]);         % adding inport
      |     add_block('DAEMOT_Lib/Support Functions/Sink',[blk,'/Sink',num2str(i)],'Position',[745 i*80-14 810 i*80+14]);         % adding inport
      |     add_block('simulink/Signal Routing/From',      [blk,'/pout',num2str(i)],    'Position',[625 i*80-14 705 i*80+14]);         % adding inport
      |     add_block('simulink/Signal Routing/From',       [blk,'/min',num2str(i)],     'Position',[935 -258+i*20 1015 -242+i*20]);         % adding inport
      |     add_block('simulink/Signal Routing/From',       [blk,'/tin',num2str(i)],     'Position',[935 1+i*20 1015 19+i*20]);         % adding inport
      |     
      |     % set goto and from tags
      |     set_param([blk,'/gm',num2str(i)],'GotoTag',char(horzcat('M_in',num2str(i))))
      |     set_param([blk,'/gt',num2str(i)],'GotoTag',char(horzcat('T_in',num2str(i))))
      |     %set_param([blk,'/gp',num2str(i)],'GotoTag',char(horzcat('P_in',num2str(i))))
      |     set_param([blk,'/pout',num2str(i)],'GotoTag',char('P'))
      |     set_param([blk,'/min',num2str(i)],'GotoTag',char(horzcat('M_in',num2str(i))))
      |     set_param([blk,'/tin',num2str(i)],'GotoTag',char(horzcat('T_in',num2str(i))))
      |     
      |     % set goto and from background colors
      |     set_param([blk,'/gm',num2str(i)],'BackgroundColor','yellow')
      |     set_param([blk,'/gt',num2str(i)],'BackgroundColor','yellow')
      |     %set_param([blk,'/gp',num2str(i)],'BackgroundColor','yellow')
      |     set_param([blk,'/min',num2str(i)],'BackgroundColor','yellow')
      |     set_param([blk,'/tin',num2str(i)],'BackgroundColor','yellow')
      |     set_param([blk,'/pout',num2str(i)],'BackgroundColor','cyan')
      |     
      |     % add lines
      |     add_line(blk,['In',num2str(i),'/1'], ['gb',num2str(i),'/1'],'AutoRouting','on')
      |     add_line(blk,['gb',num2str(i),'/1'],  ['gm',num2str(i),'/1'],'AutoRouting','on')
      |     add_line(blk,['gb',num2str(i),'/2'],  ['gt',num2str(i),'/1'],'AutoRouting','on')
      |     add_line(blk,['gb',num2str(i),'/3'],  ['gp',num2str(i),'/1'],'AutoRouting','on')
      |     add_line(blk,['pout',num2str(i),'/1'],  ['Sink',num2str(i),'/1'],'AutoRouting','on')
      |     add_line(blk,['min',num2str(i),'/1'],  ['Mux_In_1/',num2str(i)],'AutoRouting','on')
      |     add_line(blk,['tin',num2str(i),'/1'],  ['Mux_In_3/',num2str(i)],'AutoRouting','on')
      |     
      | end
      | 
      | % generate inports, bus selectors, and route lines to each vector concat
      | for i = hblock.Ports(2)+1:str2num(hblock.n_out)
      |     
      |     % add blocks
      |     add_block('simulink/Ports & Subsystems/Out1',   [blk,'/Out',num2str(i)],   'Position',[30 i*80-25+20 60 i*80-12+20]);         % adding inport
      |     add_block('simulink/Signal Routing/From',       [blk,'/m',num2str(i)],     'Position',[-150 i*80-20 -70 i*80-2]);         % adding inport
      |     add_block('simulink/Signal Routing/From',       [blk,'/t',num2str(i)],     'Position',[-150 i*80-20+20 -70 i*80-2+20]);         % adding inport
      |     add_block('simulink/Signal Routing/From',       [blk,'/p',num2str(i)],     'Position',[-150 i*80-20+40 -70 i*80-2+40]);         % adding inport
      |     add_block('simulink/Signal Routing/Bus Creator',[blk,'/b',num2str(i)],     'Position',[5 i*80-20+20-18 10 i*80-2+20+2]);         % adding inport
      |     add_block('DAEMOT_Lib/Support Functions/Source',[blk,'/Source',num2str(i)],'Position',[395 i*80-14 460 i*80+14]);         % adding inport
      |     add_block('simulink/Signal Routing/Goto',       [blk,'/g',num2str(i)],     'Position',[505 i*80-9 585 i*80+9]);         % adding inport
      |     add_block('simulink/Signal Routing/From',       [blk,'/mout',num2str(i)],  'Position',[935 -129+i*20 1015 -111+i*20]);         % adding inport
      |     %add_block('simulink/Signal Routing/Goto',      [blk,'/tout',num2str(i)],   'Position',[1455 -259+i*20 1535 -241+i*20]);         % adding inport
      |     
      |     % set goto and from tags
      |     set_param([blk,'/m',num2str(i)],'GotoTag',char(horzcat('M_out',num2str(i))))
      |     %set_param([blk,'/t',num2str(i)],'GotoTag',char(horzcat('T_out',num2str(i))))
      |     set_param([blk,'/t',num2str(i)],'GotoTag',char('T'))
      |     set_param([blk,'/p',num2str(i)],'GotoTag',char('P'))
      |     set_param([blk,'/g',num2str(i)],'GotoTag',char(horzcat('M_out',num2str(i))))
      |     set_param([blk,'/mout',num2str(i)],'GotoTag',char(horzcat('M_out',num2str(i))))
      |     %set_param([blk,'/tout',num2str(i)],'GotoTag',char(horzcat('T_out',num2str(i))))
      |     set_param([blk,'/b',num2str(i)],'Inputs','3')
      |     
      |     % set goto and from background colors
      |     set_param([blk,'/t',num2str(i)],'BackgroundColor','cyan')
      |     set_param([blk,'/m',num2str(i)],'BackgroundColor','cyan')
      |     set_param([blk,'/p',num2str(i)],'BackgroundColor','cyan')
      |     set_param([blk,'/g',num2str(i)],'BackgroundColor','cyan')
      |     set_param([blk,'/mout',num2str(i)],'BackgroundColor','cyan')
      |     %set_param([blk,'/tout',num2str(i)],'BackgroundColor','cyan')
      |     
      |     % add lines
      |     add_line(blk,['m',num2str(i),'/1'],['b',num2str(i),'/1'],'AutoRouting','on')
      |     p = get_param([blk,'/m',num2str(i)],'PortHandles');
      |     l = get_param(p.Outport,'Line');
      |     set_param(l,'Name','mdot_kgps')
      |     
      |     add_line(blk,['t',num2str(i),'/1'],['b',num2str(i),'/2'],'AutoRouting','on')
      |     p = get_param([blk,'/t',num2str(i)],'PortHandles');
      |     l = get_param(p.Outport,'Line');
      |     set_param(l,'Name','T_C')
      |     
      |     add_line(blk,['p',num2str(i),'/1'],['b',num2str(i),'/3'],'AutoRouting','on')
      |     p = get_param([blk,'/p',num2str(i)],'PortHandles');
      |     l = get_param(p.Outport,'Line');
      |     set_param(l,'Name','P_kPa')
      |     
      |     add_line(blk,['b',num2str(i),'/1'],['Out',num2str(i),'/1'],'AutoRouting','on')
      |     add_line(blk,['Source',num2str(i),'/1'],['g',num2str(i),'/1'],'AutoRouting','on')
      |     add_line(blk,['mout',num2str(i),'/1'],  ['Mux_In_2/',num2str(i)],'AutoRouting','on')
      |     %add_line(blk,['Mux_Out_1/',num2str(i)], ['tout',num2str(i),'/1'],'AutoRouting','on')
      | end
      | 
      | try
      |     set_param([blk,'/Selector1'],'InputPortWidth',num2str(hblock.n_in))
      |     set_param([blk,'/Selector2'],'InputPortWidth',num2str(hblock.n_in))
      |     
      |     selector_str = '[1 ';
      |     for i = 2:str2num(hblock.n_in)
      |         selector_str = [selector_str,num2str(i),' '];
      |     end
      |     selector_str = [selector_str,']'];
      |     set_param([blk,'/Selector1'],'IndexParamArray',{selector_str})%num2cell(1:hblock.n_in))
      |     set_param([blk,'/Selector2'],'IndexParamArray',{selector_str})%num2cell(1:hblock.n_in))
      | catch
      |     selector_str = '[1 ';
      |     for i = 2:str2num(hblock.n_in)
      |         selector_str = [selector_str,num2str(i),' '];
      |     end
      |     selector_str = [selector_str,']'];
      |     set_param([blk,'/Selector1'],'IndexParamArray',{selector_str})%num2cell(1:hblock.n_in))
      |     set_param([blk,'/Selector2'],'IndexParamArray',{selector_str})%num2cell(1:hblock.n_in))
      |     
      |     set_param([blk,'/Selector1'],'InputPortWidth',num2str(hblock.n_in))
      |     set_param([blk,'/Selector2'],'InputPortWidth',num2str(hblock.n_in))
      | end 
      |     
      |     clear h blk hblock
      settings: CopyFcn=|
      | h      = get_param(gcb,'handle');   % Get block handle
      | blk    = gcb;
      | 
      | set_param(blk, 'LinkStatus', 'inactive')
      settings: OpenFcn=|
      | load('Fluids.mat');
      | Set_Fluid_Popup_Names( Fluid )
      mask TypeOptions fluid: Fuel | Water | Air | PG50
      mask DialogControl Container4 Prompt: Parameters
      mask DialogControl Container12 Prompt: Nonlinear Model
      mask DialogControl Container15 Prompt: Component Sizing - Nominal Values
      mask Display:
      | image(imread('Split.jpg'));
      | 
      | text(0.5,0.95,['{\bf',fluid,' Split/Junction}'],'TexMode','on','horizontalAlignment', 'center')
      | text(0.5,0.08,['{(P)}'],'TexMode','on','horizontalAlignment', 'center')
      | 
      | h      = get_param(gcb,'handle');   % Get block handle
      | blk    = gcb;
      | hblock = get(h);     % Parse out handles structure
      | for i = 1:str2num(hblock.n_in)
      |     port_label('input',i,horzcat('Flow In #',num2str(i)))
      | end
      | for i = 1:str2num(hblock.n_out)
      |     port_label('output',i,horzcat('Flow Out #',num2str(i)))
      | end
  Junction1 : Subsystem  AncestorBlock=DAEMOT_Lib/Thermal/Flow Split_Junction  mask(Split/Junction){fluid=PG50, n_out=2, n_in=1, cp_f=110, T_init=22, D=0.013, L=0.1, t=0.0015, E=2.4e6, v=0.4}
      mask prompts: fluid "Fluid Type"; n_out "Number of Outlet Flows"; n_in "Number of Inlet Flows"; cp_f "specific heat"; T_init "Initial Temperature [°C]"; D "Diameter [m]"; L "Length [m]"; t "Tube Wall Thickness [m]"; E "Tube Modulus of Elasticity [kPa]"; v "Tube Poisson Ratio [-]"
      mask help: Splits and junctions flows using dynamic relationships. Note that the library link of the block is disabled when it is imported into a model.
      mask init: same as ToySystem/Junction
      settings: CopyFcn=|
      | h      = get_param(gcb,'handle');   % Get block handle
      | blk    = gcb;
      | 
      | set_param(blk, 'LinkStatus', 'inactive')
      settings: OpenFcn=|
      | load('Fluids.mat');
      | Set_Fluid_Popup_Names( Fluid )
      mask TypeOptions fluid: Fuel | Water | Air | PG50
      mask DialogControl Container4 Prompt: Parameters
      mask DialogControl Container12 Prompt: Nonlinear Model
      mask DialogControl Container15 Prompt: Component Sizing - Nominal Values
      mask Display:
      | image(imread('Split.jpg'));
      | 
      | text(0.5,0.95,['{\bf',fluid,' Split/Junction}'],'TexMode','on','horizontalAlignment', 'center')
      | text(0.5,0.08,['{(P)}'],'TexMode','on','horizontalAlignment', 'center')
      | 
      | h      = get_param(gcb,'handle');   % Get block handle
      | blk    = gcb;
      | hblock = get(h);     % Parse out handles structure
      | for i = 1:str2num(hblock.n_in)
      |     port_label('input',i,horzcat('Flow In #',num2str(i)))
      | end
      | for i = 1:str2num(hblock.n_out)
      |     port_label('output',i,horzcat('Flow Out #',num2str(i)))
      | end
  Tank 1 : Subsystem  AncestorBlock=DAEMOT_Lib/Thermal/Multi-Port Fluid Tank  mask(Multi-Port Fluid Tank){fluid=PG50, T_init=22, m_init=1.0433, P_init=103.0361, cp_f=22}
      mask prompts: fluid "Fluid Type"; T_init "Initial Fluid Temperature [°C]"; m_init "Initial Fluid Mass [kg] (fcn of height)"; P_init "Initial Fluid Pressure [kPa] (fcn of height)"; cp_f "SpecificHeat"
      mask help: Tracks the time rate of change for fluid mass and temperature, allowing for multiple inlet and outlet flows.
      settings: CopyFcn=|
      | h      = get_param(gcb,'handle');   % Get block handle
      | blk    = gcb;
      | 
      | set_param(blk, 'LinkStatus', 'inactive')
      settings: OpenFcn=|
      | load('Fluids.mat');
      | Set_Fluid_Popup_Names( Fluid )
      mask TypeOptions fluid: Fuel | Water | Air | PG50
      mask DialogControl Container8 Prompt: Parameters
      mask Display:
      | image(imread('Res.jpg'))
      | 
      | text(0.5,0.95,['{\bf ',fluid,' Multi-Port Tank}'],'TexMode','on','horizontalAlignment', 'center')
      | text(0.5,0.08,['{(P)}'],'TexMode','on','horizontalAlignment', 'center')
      | 
      | port_label('input',1,'Flow In')
      | port_label('input',2,'Amb. Temp. [°C]')
      | port_label('output',1,'Flow Out')
      | 
      | % h      = get_param(gcb,'handle');   % Get block handle
      | % blk    = gcb;
      | % hblock = get(h);     % Parse out handles structure
      | % for i = 1:str2num(hblock.Num_In)
      | %     port_label('input',i,horzcat('Flow In #',num2str(i)))
      | % end
      | % port_label('input',str2num(hblock.Num_In)+1,'Amb. Temp. [°C]')
      | % for i = 1:str2num(hblock.Num_Out)
      | %     port_label('output',i,horzcat('Flow Out #',num2str(i)))
      | % end
  Tank 2 : Subsystem  AncestorBlock=DAEMOT_Lib/Thermal/Multi-Port Fluid Tank  mask(Multi-Port Fluid Tank){fluid=PG50, T_init=22, m_init=1.0433, P_init=103.0361, cp_f=22}
      mask prompts: fluid "Fluid Type"; T_init "Initial Fluid Temperature [°C]"; m_init "Initial Fluid Mass [kg] (fcn of height)"; P_init "Initial Fluid Pressure [kPa] (fcn of height)"; cp_f "SpecificHeat"
      mask help: Tracks the time rate of change for fluid mass and temperature, allowing for multiple inlet and outlet flows.
      settings: CopyFcn=|
      | h      = get_param(gcb,'handle');   % Get block handle
      | blk    = gcb;
      | 
      | set_param(blk, 'LinkStatus', 'inactive')
      settings: OpenFcn=|
      | load('Fluids.mat');
      | Set_Fluid_Popup_Names( Fluid )
      mask TypeOptions fluid: Fuel | Water | Air | PG50
      mask DialogControl Container8 Prompt: Parameters
      mask Display:
      | image(imread('Res.jpg'))
      | 
      | text(0.5,0.95,['{\bf ',fluid,' Multi-Port Tank}'],'TexMode','on','horizontalAlignment', 'center')
      | text(0.5,0.08,['{(P)}'],'TexMode','on','horizontalAlignment', 'center')
      | 
      | port_label('input',1,'Flow In')
      | port_label('input',2,'Amb. Temp. [°C]')
      | port_label('output',1,'Flow Out')
      | 
      | % h      = get_param(gcb,'handle');   % Get block handle
      | % blk    = gcb;
      | % hblock = get(h);     % Parse out handles structure
      | % for i = 1:str2num(hblock.Num_In)
      | %     port_label('input',i,horzcat('Flow In #',num2str(i)))
      | % end
      | % port_label('input',str2num(hblock.Num_In)+1,'Amb. Temp. [°C]')
      | % for i = 1:str2num(hblock.Num_Out)
      | %     port_label('output',i,horzcat('Flow Out #',num2str(i)))
      | % end
  wires:
  Tank 1/1(Out1) -> Cold Plate/1(In1)
  Cold Plate/1(Out1) -> Junction/1(In1)
  Tank 2/1(Out1) -> Junction/2(In2)
  Junction/1(Out1) -> HX/2(In2)
  Junction1/1(Out1) -> Tank 1/1(In1)
  Junction1/2(Out2) -> Tank 2/1(In1)
  HX/2(Out2) -> Junction1/1(In1)
  HX/1(Out1) -> Generic Sink/1(In1)
  Generic Source/1(Out1) -> HX/1(In1)
  Generic Source1/1(Out1) -> Cold Plate/2(Q)
  Generic Source2/1(Out1) -> Tank 1/2(Q)
  Generic Source3/1(Out1) -> Tank 2/2(Q)
